simulink model "slexBistaticExample"  (R2024b)
settings: Solver=FixedStepDiscrete  StartTime=0.0  StopTime=0.16384  RelTol=1e-3  EnableMultiTasking=on
PreLoadFcn:
  | helperslexBistaticParam
undefined symbols (not defined in the file or in its folder): paramBistatic, parula
libraries: phasedenvlib x6, phasedtxrxlib x2, dspstat3 x2, phasedwavlib x1, phaseddetectlib x1, dspobslib x1, dspmathops x1, phasedmisclib x1
CloseFcn:
  | clear paramBistatic
settings Model: Creator=The MathWorks, Inc.  LastModifiedBy=ayush
settings SolverCC: AlgebraicLoopSolver=TrustRegion  MaxZcPerStep=1
settings DataIOCC: LimitDataPoints=on  SaveFormat=Array  ReturnWorkspaceOutputs=off
settings OptimizationCC: LifeSpan=inf
settings DebuggingCC: ReadBeforeWriteMsg=DisableAll  WriteAfterWriteMsg=DisableAll  WriteAfterReadMsg=DisableAll  SolverPrmCheckMsg=warning  MultiTaskDSMMsg=none  UnconnectedInputMsg=warning  UnconnectedOutputMsg=warning  UnconnectedLineMsg=warning  AllowSymbolicDim=off  SFUnexpectedBacktrackingDiag=warning  SFNoUnconditionalDefaultTransitionDiag=warning  SFExecutionAtInitializationDiag=none  ArithmeticOperatorsInVariantConditions=warning
settings HardwareCC: ProdBitPerPointer=32  ProdBitPerSizeT=32  ProdBitPerPtrDiffT=32  ProdLargestAtomicFloat=None  ProdIntDivRoundTo=Undefined  ProdEndianess=Unspecified  ProdWordSize=32  ProdHWDeviceType=32-bit Generic
settings ModelReferenceCC: UpdateModelReferenceTargets=IfOutOfDate  EnableRefExpFcnMdlSchedulingChecks=on  PropagateSignalLabelsOutOfModel=off
settings SFSimCC: SFSimEcho=off  SimUseLocalCustomCode=off  CustomCodeUndefinedFunction=UseInterfaceOnly
settings RTWCC: RTWUseLocalCustomCode=off  GPUComputeCapability=3.5
settings CodeAppCC: StateflowObjectComments=on
settings GRTTargetCC: TargetLangStandard=C89/C90 (ANSI)
settings ConfigComp: CovMetricSettings=dw  CovSaveCumulativeToWorkspaceVar=on  CovSaveSingleToWorkspaceVar=on  CovExternalEMLEnable=off  CovSFcnEnable=off

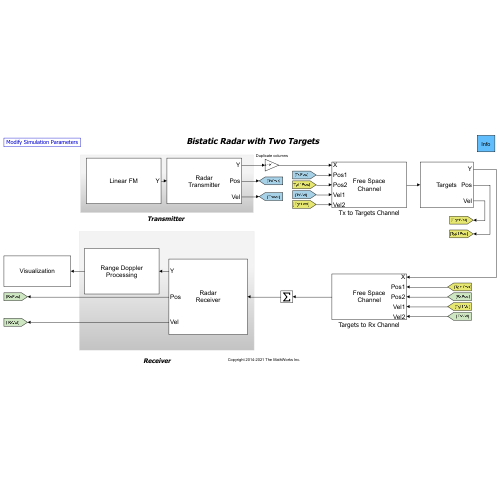
[thumbnail: Simulink's stored preview of the top-level diagram]
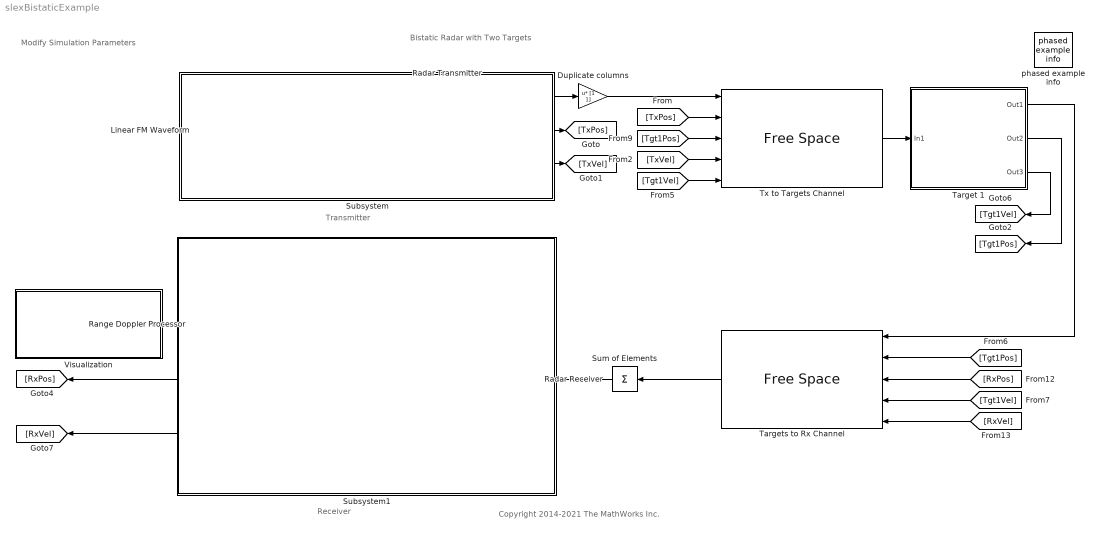
== system slexBistaticExample ==
  note: Transmitter
  note: Copyright 2014-2021 The MathWorks Inc.
  note: Bistatic Radar with Two Targets
  note: Receiver
  note: Modify Simulation Parameters
  Duplicate columns : Gain  Gain=[1 1]  Multiplication=Matrix(u*K)
  Linear FM Waveform : phasedwavlib/Linear FM Waveform  SampleRate=paramBistatic.Fs  DurationSpecification=Pulse width  PulseWidth=paramBistatic.tau  DutyCycle=0.5  PRF=paramBistatic.PRF  PRFSelectionInputPort=off  SimulationTimeSource=Derive from waveform parameters  SweepBandwidth=paramBistatic.bw  SweepDirection=Up  SweepInterval=Positive  Envelope=Rectangular  FrequencyOffsetSource=Property  FrequencyOffset=0  OutputFormat=Pulses  NumSamples=100  NumPulses=1  PRFOutputPort=off  CoefficientsOutputPort=off  SimulateUsing=Interpreted execution
  Radar Receiver : Subsystem
      mask Display:
      | disp('Radar\nReceiver')
      | port_label('output',1,'Y')
      | port_label('output',2,'Pos')
      | port_label('output',3,'Vel')
  Radar Transmitter : Subsystem
      mask Display:
      | disp('Radar\nTransmitter')
      | port_label('output',1,'Y')
      | port_label('output',2,'Pos')
      | port_label('output',3,'Vel')
  Range Doppler Processor : Subsystem
      mask Display: disp('Range Doppler\nProcessing')
  Subsystem : Subsystem
  Subsystem1 : Subsystem
  Sum of Elements : Sum  Inputs=+  CollapseMode=Specified dimension  CollapseDim=2
  Target 1 : Subsystem
      mask Display:
      | disp('Targets')
      | port_label('output',1,'Y')
      | port_label('output',2,'Pos')
      | port_label('output',3,'Vel')
  Targets to Rx Channel : phasedenvlib/Free Space  PropagationSpeed=paramBistatic.pspeed  OperatingFrequency=paramBistatic.Fc  TwoWayPropagation=off  SampleRateFromInputCheckbox=on  SampleRate=1e6  MaximumDistanceSource=Property  MaximumDistance=paramBistatic.MaxRange  MaximumNumInputSamplesSource=Auto  MaximumNumInputSamples=1000  SimulateUsing=Interpreted execution
  Tx to Targets Channel : phasedenvlib/Free Space  PropagationSpeed=paramBistatic.pspeed  OperatingFrequency=paramBistatic.Fc  TwoWayPropagation=off  SampleRateFromInputCheckbox=on  SampleRate=1e6  MaximumDistanceSource=Property  MaximumDistance=paramBistatic.MaxRange  MaximumNumInputSamplesSource=Auto  MaximumNumInputSamples=1000  SimulateUsing=Interpreted execution
  Visualization : Subsystem
      mask Display: disp('Visualization')
  phased example info : phasedmisclib/phased example info  SystemSampleTime=-1  VariantActivationTime=update diagram  AllowFlexibleInterface=on  Latency=0  AutoFrameSizeCalculation=off
  wires:
  Target 1/1(Out1) -> Targets to Rx Channel/1
  Tx to Targets Channel/1 -> Target 1/1(In1)
  Linear FM Waveform/1 -> Radar Transmitter/1(In1)
  Radar Transmitter/1(Out1) -> Duplicate columns/1
  Radar Transmitter/2(Out2) -> [TxPos]
  Radar Transmitter/3(Out3) -> [TxVel]
  Target 1/2(Out2) -> [Tgt1Pos]
  Target 1/3(Out3) -> [Tgt1Vel]
  Radar Receiver/2(Out2) -> [RxPos]
  Radar Receiver/3(Out3) -> [RxVel]
  [Tgt1Pos] -> Targets to Rx Channel/2
  [RxPos] -> Targets to Rx Channel/3
  [Tgt1Vel] -> Targets to Rx Channel/4
  [RxVel] -> Targets to Rx Channel/5
  [TxPos] -> Tx to Targets Channel/2
  [Tgt1Pos] -> Tx to Targets Channel/3
  [TxVel] -> Tx to Targets Channel/4
  [Tgt1Vel] -> Tx to Targets Channel/5
  Radar Receiver/1(Out1) -> Range Doppler Processor/1(In1)
  Range Doppler Processor/1(Out1) -> Visualization/1(In1)
  Duplicate columns/1 -> Tx to Targets Channel/1
  Sum of Elements/1 -> Radar Receiver/1(In1)
  Targets to Rx Channel/1 -> Sum of Elements/1

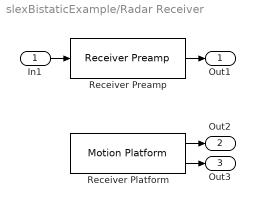
== system slexBistaticExample/Radar Receiver ==
  In1 : Inport
  Receiver Platform : phasedenvlib/Motion Platform  MotionModel=Velocity  InitialPosition=paramBistatic.RadarRxPos  InitialVelocity=[ 0; 0; 0 ]  VelocitySource=Property  Velocity=paramBistatic.RadarRxVel  AccelerationSource=Property  Acceleration=[0;0;0]  CustomTrajectory=[ 0, 0, 0, 0, 0, 0, 0; 1, 0, 0, 0, 0, 0, 0 ]  ScanMode=None  InitialScanAngle=0  AzimuthSpan=[ -60, 60 ]  AzimuthScanRate=10  InitialOrientationAxes=eye( 3 )  OrientationAxesOutputPort=off  ElapsedTimeSource=Auto  SampleRateFromInputCheckbox=on  SampleRate=1e6  SimulateUsing=Interpreted execution
  Receiver Preamp : phasedtxrxlib/Receiver Preamp  Gain=20  LossFactor=0  NoiseMethod=Noise temperature  NoiseFigure=0  ReferenceTemperature=290  SampleRateFromInputCheckbox=on  SampleRate=1e6  NoisePower=0  EnableInputPort=off  PhaseNoiseInputPort=off  SeedSource=Auto  Seed=0  SimulateUsing=Interpreted execution
  Out1 : Outport  VectorParamsAs1DForOutWhenUnconnected=off
  Out2 : Outport  Port=2  VectorParamsAs1DForOutWhenUnconnected=off
  Out3 : Outport  Port=3  VectorParamsAs1DForOutWhenUnconnected=off
  wires:
  Receiver Platform/1 -> Out2/1
  In1/1 -> Receiver Preamp/1
  Receiver Preamp/1 -> Out1/1
  Receiver Platform/2 -> Out3/1

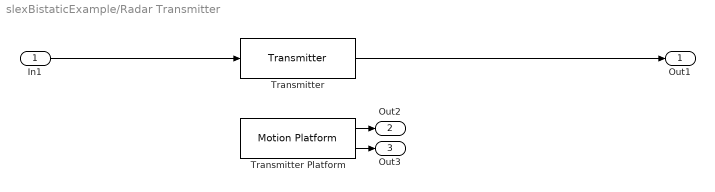
== system slexBistaticExample/Radar Transmitter ==
  In1 : Inport
  Transmitter : phasedtxrxlib/Transmitter  PeakPower=paramBistatic.ppow  GainMethod=Linear  Gain=20  LossFactor=0  OIP3=Inf  Table=[ -25, 5, -1; -10, 20, -2; 0, 27, 12; 5, 28, 12 ]  InUseOutputPort=off  CoherentOnTransmit=on  PhaseNoiseOutputPort=off  SimulateUsing=Interpreted execution  NoiseMethod=None  NoiseFigure=3  NoiseFactor=2  NoiseTemperature=290  ReferenceTemperature=290  SampleRate=1e6  SampleRateFromInputCheckbox=on  PhaseOffset=0  SeedSource=Auto  Seed=0
  Transmitter Platform : phasedenvlib/Motion Platform  MotionModel=Velocity  InitialPosition=paramBistatic.RadarTxPos  InitialVelocity=[ 0; 0; 0 ]  VelocitySource=Property  Velocity=paramBistatic.RadarTxVel  AccelerationSource=Property  Acceleration=[0;0;0]  CustomTrajectory=[ 0, 0, 0, 0, 0, 0, 0; 1, 0, 0, 0, 0, 0, 0 ]  ScanMode=None  InitialScanAngle=0  AzimuthSpan=[ -60, 60 ]  AzimuthScanRate=10  InitialOrientationAxes=eye( 3 )  OrientationAxesOutputPort=off  ElapsedTimeSource=Auto  SampleRateFromInputCheckbox=on  SampleRate=1e6  SimulateUsing=Interpreted execution
  Out1 : Outport  VectorParamsAs1DForOutWhenUnconnected=off
  Out2 : Outport  Port=2  VectorParamsAs1DForOutWhenUnconnected=off
  Out3 : Outport  Port=3  VectorParamsAs1DForOutWhenUnconnected=off
  wires:
  In1/1 -> Transmitter/1
  Transmitter Platform/1 -> Out2/1
  Transmitter Platform/2 -> Out3/1
  Transmitter/1 -> Out1/1

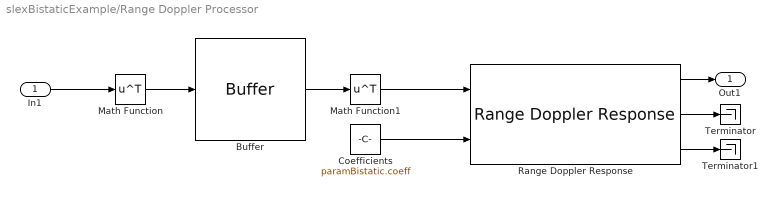
== system slexBistaticExample/Range Doppler Processor ==
  In1 : Inport
  Buffer : Buffer
  Coefficients : Constant  Value=paramBistatic.coeff
  Math Function : Math  Operator=transpose  SignedPower=on
  Math Function1 : Math  Operator=transpose  SignedPower=on
  Range Doppler Response : phaseddetectlib/Range Doppler Response  RangeMethod=Matched filter  PropagationSpeed=paramBistatic.pspeed  SampleRateFromInputCheckbox=off  SampleRate=paramBistatic.Fs  SweepSlope=1e9  DechirpInput=off  RangeFFTLengthSource=Auto  RangeFFTLength=1024  RangeWindow=None  RangeSidelobeAttenuation=30  CustomRangeWindow=@hamming  ReferenceRangeCentered=on  ReferenceRange=0  MaximumNumInputSamplesSource=Auto  MaximumNumInputSamples=100  PRFSource=Auto  PRF=10e3  DopplerFFTLengthSource=Property  DopplerFFTLength=256  DopplerWindow=Hamming  DopplerSidelobeAttenuation=30  CustomDopplerWindow=@hamming  DopplerOutput=Speed  OperatingFrequency=paramBistatic.Fc  SimulateUsing=Interpreted execution
  Terminator : Terminator
  Terminator1 : Terminator
  Out1 : Outport  VectorParamsAs1DForOutWhenUnconnected=off
  wires:
  In1/1 -> Math Function/1
  Math Function/1 -> Buffer/1
  Buffer/1 -> Math Function1/1
  Math Function1/1 -> Range Doppler Response/1
  Range Doppler Response/2 -> Terminator/1
  Range Doppler Response/3 -> Terminator1/1
  Coefficients/1 -> Range Doppler Response/2
  Range Doppler Response/1 -> Out1/1

== system slexBistaticExample/Subsystem ==

== system slexBistaticExample/Subsystem1 ==

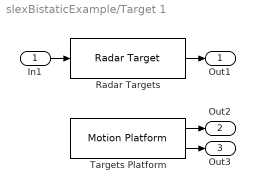
== system slexBistaticExample/Target 1 ==
  In1 : Inport
  Radar Targets : phasedenvlib/Radar Target  EnablePolarization=off  Mode=Monostatic  MeanRCSSource=Property  ScatteringMatrixSource=Property  MeanRCS=paramBistatic.RCS  ScatteringMatrix=eye( 2 )  Model=Nonfluctuating  PropagationSpeed=paramBistatic.pspeed  OperatingFrequency=paramBistatic.Fc  SeedSource=Auto  Seed=0  SimulateUsing=Interpreted execution
  Targets Platform : phasedenvlib/Motion Platform  MotionModel=Velocity  InitialPosition=paramBistatic.TargetPos  InitialVelocity=[ 0; 0; 0 ]  VelocitySource=Property  Velocity=paramBistatic.TargetVel  AccelerationSource=Property  Acceleration=[0;0;0]  CustomTrajectory=[ 0, 0, 0, 0, 0, 0, 0; 1, 0, 0, 0, 0, 0, 0 ]  ScanMode=None  InitialScanAngle=0  AzimuthSpan=[ -60, 60 ]  AzimuthScanRate=10  InitialOrientationAxes=eye( 3 )  OrientationAxesOutputPort=off  ElapsedTimeSource=Auto  SampleRateFromInputCheckbox=on  SampleRate=1e6  SimulateUsing=Interpreted execution
  Out1 : Outport  VectorParamsAs1DForOutWhenUnconnected=off
  Out2 : Outport  Port=2  VectorParamsAs1DForOutWhenUnconnected=off
  Out3 : Outport  Port=3  VectorParamsAs1DForOutWhenUnconnected=off
  wires:
  Radar Targets/1 -> Out1/1
  In1/1 -> Radar Targets/1
  Targets Platform/2 -> Out3/1
  Targets Platform/1 -> Out2/1

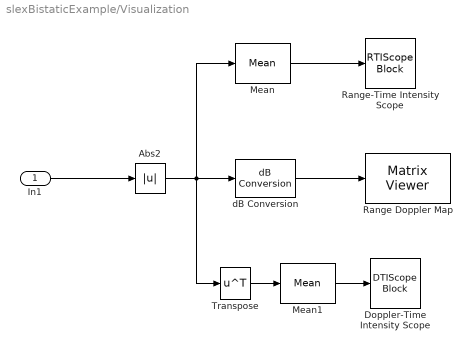
== system slexBistaticExample/Visualization ==
  In1 : Inport
  Abs2 : Abs  SaturateOnIntegerOverflow=off
  Doppler-Time Intensity Scope : DTIScopeBlock  WindowPosition=[775.000000,383.000000,393.000000,271.000000,]  ScopeFrameLocation=window  DopplerOffset=paramBistatic.dopOff  DopplerResolution=paramBistatic.dopRes  TimeSpan=paramBistatic.timeSpan  TimeResolution=paramBistatic.timeRes  ColorbarLabel=magnitude (V)  OperatingFrequency=paramBistatic.Fc  PropagationSpeed=paramBistatic.pspeed  DopplerOutput=Speed
  Mean : dspstat3/Mean  run=off  InputProcessing=Columns as channels (frame based)  reset_popup=None  directionMode=Each row  dimension=1  roiEnable=off  roiType=Rectangles  roiPortion=Entire ROI  roiOutput=Individual statistics for each ROI  roiFlag=off  roundingMode=Floor  overflowMode=off  outputDataTypeStr=Inherit: Same as accumulator  outputMin=[]  outputMax=[]  outputLastDataTypeStr=Inherit: Same as accumulator
  Mean1 : dspstat3/Mean  run=off  InputProcessing=Columns as channels (frame based)  reset_popup=None  directionMode=Each row  dimension=1  roiEnable=off  roiType=Rectangles  roiPortion=Entire ROI  roiOutput=Individual statistics for each ROI  roiFlag=off  roundingMode=Floor  overflowMode=off  outputDataTypeStr=Inherit: Same as accumulator  outputMin=[]  outputMax=[]  outputLastDataTypeStr=Inherit: Same as accumulator
  Range Doppler Map : dspobslib/Matrix Viewer  ImageParams=off  CMapStr=parula(256)  AxisColorbar=on  AxisParams=off  AxisOrigin=Upper left corner  AxisTickMode=User-defined  XTickRange=[-5625 5.6030e3]  YTickRange=[0 47950]/1000  XLabel=Speed (km/h)  YLabel=Range (km)  ZLabel=Power (dB)  FigPos=[350 403 560 420]  AxisZoom=off
      settings: YMin=-167.4215  YMax=-56.9568
  Range-Time Intensity Scope : RTIScopeBlock  WindowPosition=[775.000000,382.000000,391.000000,273.000000,]  ScopeFrameLocation=window  RangeResolution=paramBistatic.rngRes  TimeSpan=paramBistatic.timeSpan  TimeResolution=paramBistatic.timeRes  ColorbarLabel=magnitude (V)
  Transpose : Math  Operator=transpose
  dB Conversion : dspmathops/dB Conversion  dBtype=dB  intype=Amplitude  R=1  fuzz=on
  wires:
  Abs2/1 -> Transpose/1, Mean/1, dB Conversion/1
  dB Conversion/1 -> Range Doppler Map/1
  In1/1 -> Abs2/1
  Transpose/1 -> Mean1/1
  Mean/1 -> Range-Time Intensity Scope/1
  Mean1/1 -> Doppler-Time Intensity Scope/1
